simulink model "Question_10_SL"  (R2017a)
settings: Solver=VariableStepAuto  StartTime=0.0  StopTime=10.0  RelTol=1e-3
settings Model: Creator=berthj01  LastModifiedBy=vonl01

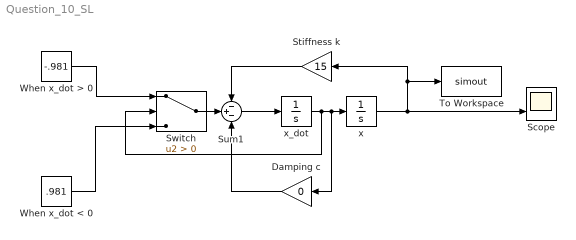
== system Question_10_SL ==
  Damping c : Gain  Gain=0
  Scope : Scope  NumInputPorts=2
  Stiffness k : Gain  Gain=15
  Sum1 : Sum  Inputs=-+-
  Switch : Switch  Criteria=u2 > Threshold  ZeroCross=off
  To Workspace : ToWorkspace  VariableName=simout  SampleTime=-1
  When x_dot < 0 : Constant  Value=.981
  When x_dot > 0 : Constant  Value=-.981
  x : Integrator  InitialCondition=.5
  x_dot : Integrator
  wires:
  Switch/1 -> Sum1/2
  Sum1/1 -> x_dot/1
  x_dot/1 -> Damping c/1, x/1, Switch/2
  Stiffness k/1 -> Sum1/1
  Damping c/1 -> Sum1/3
  x/1 -> Scope/2, Stiffness k/1, To Workspace/1
  When x_dot > 0/1 -> Switch/1
  When x_dot < 0/1 -> Switch/3
